simulink model "SF045A_HwAgSysArbn"  (R2013b)
settings: Solver=FixedStepDiscrete  SolverMode=SingleTasking  StartTime=0.0  StopTime=1  FixedStep=.002  RelTol=1e-3
values from neighbouring files (symbols this model uses):
  ARCHGLBPRM_2MILLISEC_SEC_F32 = DataDict.Constant    [SF045A_HwAgSysArbn_DataDict.m]
  ARCHGLBPRM_FLOATZEROTHD_ULS_F32 = DataDict.Constant    [SF045A_HwAgSysArbn_DataDict.m]
  ARCHGLBPRM_PIOVER180_ULS_F32 = DataDict.Constant    [SF045A_HwAgSysArbn_DataDict.m]
  CNVSECTOCNT_ULS_U32 = DataDict.Constant    [SF045A_HwAgSysArbn_DataDict.m]
  CNVTOMILLISEC_MILLISECPERCNT_F32 = DataDict.Constant    [SF045A_HwAgSysArbn_DataDict.m]
  FltInj_f32 = DataDict.Client    [SF045A_HwAgSysArbn_DataDict.m]
  FLTINJ_HWAGSYSARBN_HWAG = DataDict.Constant    [SF045A_HwAgSysArbn_DataDict.m]
  FLTINJ_HWAGSYSARBN_SERLCOMHWAG = DataDict.Constant    [SF045A_HwAgSysArbn_DataDict.m]
  HwAgCorrlnFlt = DataDict.NTC    [SF045A_HwAgSysArbn_DataDict.m]
  HwAgSnsrlsThdExcdd = DataDict.NTC    [SF045A_HwAgSysArbn_DataDict.m]
  HwAgSysArbnHwAgConf1Snsr = DataDict.Calibration    [SF045A_HwAgSysArbn_DataDict.m]
  HwAgSysArbnHwAgConf2Snsr = DataDict.Calibration    [SF045A_HwAgSysArbn_DataDict.m]
  HwAgSysArbnHwAgConfNoSnsr = DataDict.Calibration    [SF045A_HwAgSysArbn_DataDict.m]
  HwAgSysArbnHwAgCorrdCorrlnThd = DataDict.Calibration    [SF045A_HwAgSysArbn_DataDict.m]
  HwAgSysArbnHwAgCorrlnFailDebStep = DataDict.Calibration    [SF045A_HwAgSysArbn_DataDict.m]
  HwAgSysArbnHwAgCorrlnPassDebStep = DataDict.Calibration    [SF045A_HwAgSysArbn_DataDict.m]
  HwAgSysArbnHwAgCorrlnRng = DataDict.Calibration    [SF045A_HwAgSysArbn_DataDict.m]
  HwAgSysArbnHwAgSlewRate = DataDict.Calibration    [SF045A_HwAgSysArbn_DataDict.m]
  HwAgSysArbnHwAgSnsrlsCorrlnThd = DataDict.Calibration    [SF045A_HwAgSysArbn_DataDict.m]
  HwAgSysArbnHwAgSnsrlsKineThd = DataDict.Calibration    [SF045A_HwAgSysArbn_DataDict.m]
  HwAgSysArbnHwAgToMotAgCorrlnElpdTiLim = DataDict.Calibration    [SF045A_HwAgSysArbn_DataDict.m]
  HwAgSysArbnSerlComHwAgCorrdConf = DataDict.Calibration    [SF045A_HwAgSysArbn_DataDict.m]
  HwAgSysArbnSerlComHwAgSnsrlsConf = DataDict.Calibration    [SF045A_HwAgSysArbn_DataDict.m]
  HwAgSysArbnSlewRateTmr = DataDict.Calibration    [SF045A_HwAgSysArbn_DataDict.m]
  HWAGTHD_ULS_FLOAT32 = DataDict.Constant    [SF045A_HwAgSysArbn_DataDict.m]
  INVLDSRC_CNT_S08 = DataDict.Constant    [SF045A_HwAgSysArbn_DataDict.m]
  LRGSLEW_HWDEGPERSEC_F32 = DataDict.Constant    [SF045A_HwAgSysArbn_DataDict.m]
  NODEBSTEP_CNT_U16 = DataDict.Constant    [SF045A_HwAgSysArbn_DataDict.m]
  SLEWINPROGS_CNT_LGC = DataDict.Constant    [SF045A_HwAgSysArbn_DataDict.m]
  SLEWNOTINPROGS_CNT_LGC = DataDict.Constant    [SF045A_HwAgSysArbn_DataDict.m]
  SNSRDATASRCSELD_CNT_S08 = DataDict.Constant    [SF045A_HwAgSysArbn_DataDict.m]
  SNSRLSDATASRCSELD_CNT_S08 = DataDict.Constant    [SF045A_HwAgSysArbn_DataDict.m]
  SysGlbPrmSysKineRat = DataDict.ImprtdCal    [SF045A_HwAgSysArbn_DataDict.m]
  SysGlbPrmTorsBarStfn = DataDict.ImprtdCal    [SF045A_HwAgSysArbn_DataDict.m]
  ZEROTMR_MILLISEC_F32 = DataDict.Constant    [SF045A_HwAgSysArbn_DataDict.m]
undefined symbols (not defined in the file or in its folder): NtcSts1
libraries: NxtrLim x11, simulink x6, NxtrAbslt x6, Fil x3, autosarlib x2
(part 4 of 6)

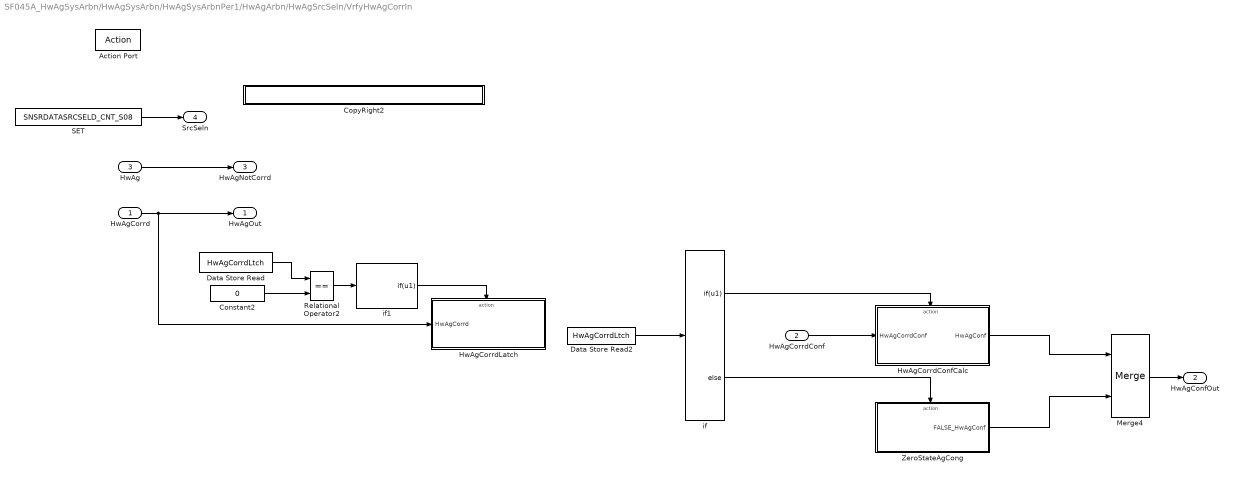
== system SF045A_HwAgSysArbn/HwAgSysArbn/HwAgSysArbnPer1/HwAgArbn/HwAgSrcSeln/VrfyHwAgCorrln ==
  HwAgCorrd : Inport
  HwAgCorrdConf : Inport  Port=2
  HwAg : Inport  Port=3
  Action Port : ActionPort  ActionType=then
  Constant2 : Constant  RequirementInfo={} %GIDa_6d460884_eb57_4a18_b5a0_8df804c20e72  Value=0  OutDataTypeStr=boolean
  CopyRight2 : Subsystem  Description=|  mask(Copyright Information){none=on}
      | Copyright info block.                                               
      |                                                                     
      | Place copyright information at the top of every subsystem in design.
      mask prompts: none "No parameters"
      mask help: Place copyright information at the top of every subsystem in design.
      mask Display:
      | NxtrConf = 'Nexteer Confidential';
      | 
      | sys = bdroot; %handle for the current model ("system")
      | first = get_param(sys,'Created');
      | first = first(end-3:end);  %year is last four digits
      | 
      | last = get_param(sys,'LastModifiedDate');
      | if isempty(last)
      |     last = datestr(now,'yyyy');
      | else
      |     last = last(end-3:end);
      | end
      | 
      | if strcmp(first,last)
      |     fprintf('%s -- Copyright %s Nexteer',NxtrConf,first)
      | else
      |     fprintf('%s -- %s%s- %s Nexteer',NxtrConf,char(169),first,last)
      | end
  Data Store Read : DataStoreRead  RequirementInfo="{'linktype_rmi_doors' '00012ce0 (/E-STEER Core/SubSystem Specifications/Application Functions - EA4/SF045A Handwheel Angle System Arbitration)' '#SF045A_137' 'true' 'REQ:  SF045A_137' '' } %GIDa_194e0ab0_9977_4834_b3f7_b4363b23e19d"  Priority=1  DataStoreName=HwAgCorrdLtch
      settings: AttributesFormatString=Priority%<priority>
  Data Store Read2 : DataStoreRead  RequirementInfo={} %GIDa_535fb5ef_e4a1_4c16_a074_9bb7e8df7af0  Priority=3  DataStoreName=HwAgCorrdLtch
      settings: AttributesFormatString=Priority%<priority>
  HwAgCorrdConfCalc : Subsystem  RequirementInfo="{'linktype_rmi_doors' '00012ce0 (/E-STEER Core/SubSystem Specifications/Application Functions - EA4/SF045A Handwheel Angle System Arbitration)' '#SF045A_143' 'true' 'REQ:  SF045A_143' '' } %GIDa_a84d203b_e366_4371_b9d3_fcddeb517755"  TreatAsAtomicUnit=on
  HwAgCorrdLatch : Subsystem  RequirementInfo="{'linktype_rmi_doors' '00012ce0 (/E-STEER Core/SubSystem Specifications/Application Functions - EA4/SF045A Handwheel Angle System Arbitration)' '#SF045A_142' 'true' 'REQ:  SF045A_142' '' } %GIDa_ab6e831f_d956_473f_8c78_8f53a50bb366"  TreatAsAtomicUnit=on
  Merge4 : Merge  RequirementInfo="{'linktype_rmi_doors' '00012ce0 (/E-STEER Core/SubSystem Specifications/Application Functions - EA4/SF045A Handwheel Angle System Arbitration)' '#SF045A_143' 'true' 'REQ:  SF045A_143' '' ; 'linktype_rmi_doors' '00012ce0 (/E-STEER Core/SubSystem Specifications/Application Functions - EA4/SF045A Handwheel Angle System Arbitration)' '#SF045A_144' 'true' 'REQ:  SF045A_144' '' } %GIDa_b0bab756_8967_46e8_af28_b116f083f0b6"
  Relational Operator2 : RelationalOperator  RequirementInfo={} %GIDa_95e6dac5_bd55_489b_9cc0_b27c478194ec  Operator===  OutDataTypeStr=boolean
  SET : Constant  Value=SNSRDATASRCSELD_CNT_S08
  ZeroStateAgCong : Subsystem  RequirementInfo="{'linktype_rmi_doors' '00012ce0 (/E-STEER Core/SubSystem Specifications/Application Functions - EA4/SF045A Handwheel Angle System Arbitration)' '#SF045A_144' 'true' 'REQ:  SF045A_144' '' } %GIDa_147c3664_39c2_4941_af40_1c56d56f150e"  TreatAsAtomicUnit=on
  if : If  RequirementInfo={} %GIDa_fd8cff81_1f47_4227_b831_50dd22e8a047  IfExpression=u1
  if1 : If  RequirementInfo={} %GIDa_17c9a915_b2cf_43c8_a6ee_d6c1fe1a00d4  IfExpression=u1  ShowElse=off
  HwAgOut : Outport
  HwAgConfOut : Outport  Port=2
  "HwAgNotCorrd " : Outport  Port=3
  SrcSeln : Outport  Port=4
  wires:
  HwAg/1 -> "HwAgNotCorrd "/1
  SET/1 -> SrcSeln/1
  HwAgCorrdConf/1 -> HwAgCorrdConfCalc/1(HwAgCorrdConf)
  Merge4/1 -> HwAgConfOut/1
  Data Store Read/1 -> Relational Operator2/1
  Constant2/1 -> Relational Operator2/2
  Data Store Read2/1 -> if/1
  if/2 -> ZeroStateAgCong/Action
  ZeroStateAgCong/1(FALSE_HwAgConf) -> Merge4/2
  if/1 -> HwAgCorrdConfCalc/Action
  HwAgCorrdConfCalc/1(HwAgConf) -> Merge4/1
  HwAgCorrd/1 -> HwAgCorrdLatch/1(HwAgCorrd), HwAgOut/1
  Relational Operator2/1 -> if1/1
  if1/1 -> HwAgCorrdLatch/Action

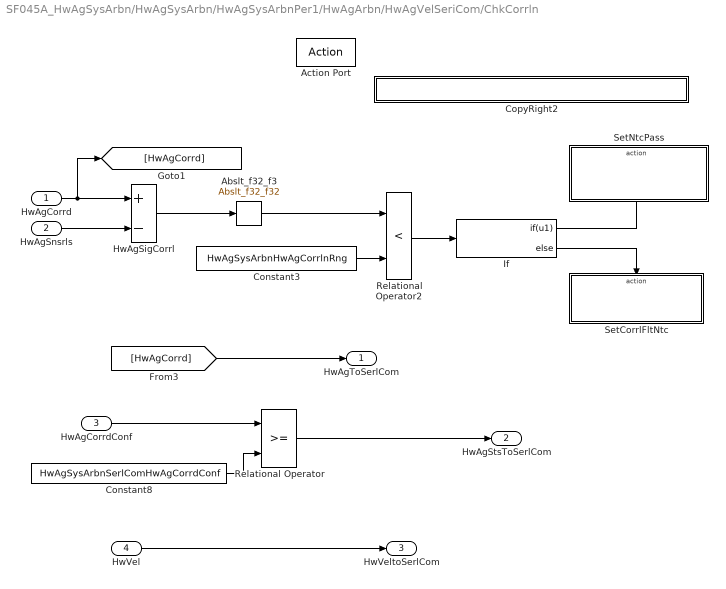
== system SF045A_HwAgSysArbn/HwAgSysArbn/HwAgSysArbnPer1/HwAgArbn/HwAgVelSeriCom/ChkCorrln ==
  HwAgCorrd : Inport
  HwAgSnsrls : Inport  Port=2
  HwAgCorrdConf : Inport  Port=3
  HwVel : Inport  Port=4
  Action Port : ActionPort  ActionType=then
  Abslt_f32_f3 : NxtrAbslt/Abslt_f32_f32  RequirementInfo={} %GIDa_00167e91_613e_4759_885d_9314db63fdd0  SFunctionSpec=single y1 = Abslt_f32_f32(single u1)
      settings: AttributesFormatString=%<Name>
  Constant3 : Constant  RequirementInfo={} %GIDa_be4a7688_2be7_4fe3_8e3d_8bacae0f8621  Value=HwAgSysArbnHwAgCorrlnRng
  Constant8 : Constant  RequirementInfo={} %GIDa_01f8480a_5c21_4e31_ac39_b28c91927747  Value=HwAgSysArbnSerlComHwAgCorrdConf
  CopyRight2 : Subsystem  Description=|  mask(Copyright Information){none=on}
      | Copyright info block.                                               
      |                                                                     
      | Place copyright information at the top of every subsystem in design.
      mask prompts: none "No parameters"
      mask help: Place copyright information at the top of every subsystem in design.
      mask Display:
      | NxtrConf = 'Nexteer Confidential';
      | 
      | sys = bdroot; %handle for the current model ("system")
      | first = get_param(sys,'Created');
      | first = first(end-3:end);  %year is last four digits
      | 
      | last = get_param(sys,'LastModifiedDate');
      | if isempty(last)
      |     last = datestr(now,'yyyy');
      | else
      |     last = last(end-3:end);
      | end
      | 
      | if strcmp(first,last)
      |     fprintf('%s -- Copyright %s Nexteer',NxtrConf,first)
      | else
      |     fprintf('%s -- %s%s- %s Nexteer',NxtrConf,char(169),first,last)
      | end
  HwAgSigCorrl : Sum  RequirementInfo="{'linktype_rmi_doors' '00012ce0 (/E-STEER Core/SubSystem Specifications/Application Functions - EA4/SF045A Handwheel Angle System Arbitration)' '#SF045A_105' 'true' 'REQ:  SF045A_105' '' } %GIDa_a5ccc499_f9e1_47ad_be00_f3d80d727547"  Inputs=+-
  If : If  IfExpression=u1
  Relational Operator : RelationalOperator  RequirementInfo="{'linktype_rmi_doors' '00012ce0 (/E-STEER Core/SubSystem Specifications/Application Functions - EA4/SF045A Handwheel Angle System Arbitration)' '#SF045A_87' 'true' 'REQ:  SF045A_87' '' } %GIDa_d7bb18e9_c0e4_41eb_b2f7_98e90d887605"  OutDataTypeStr=boolean
  Relational Operator2 : RelationalOperator  RequirementInfo="{'linktype_rmi_doors' '00012ce0 (/E-STEER Core/SubSystem Specifications/Application Functions - EA4/SF045A Handwheel Angle System Arbitration)' '#SF045A_105' 'true' 'REQ:  SF045A_105' '' } %GIDa_d5b01a50_0204_46bb_9aa8_dacdb52ec4dd"  Operator=<  OutDataTypeStr=boolean
  SetCorrlFltNtc : Subsystem  RequirementInfo="{'linktype_rmi_doors' '00012ce0 (/E-STEER Core/SubSystem Specifications/Application Functions - EA4/SF045A Handwheel Angle System Arbitration)' '#SF045A_119' 'true' 'REQ:  SF045A_119' '' ; 'linktype_rmi_doors' '00012ce0 (/E-STEER Core/SubSystem Specifications/Application Functions - EA4/SF045A Handwheel Angle System Arbitration)' '#SF045A_102' 'true' 'REQ:  SF045A_102' '' } %GIDa_ccc8f525_72d3_4104_894c_6ee731a3d477"  TreatAsAtomicUnit=on
  SetNtcPass : Subsystem  RequirementInfo="{'linktype_rmi_doors' '00012ce0 (/E-STEER Core/SubSystem Specifications/Application Functions - EA4/SF045A Handwheel Angle System Arbitration)' '#SF045A_118' 'true' 'REQ:  SF045A_118' '' ; 'linktype_rmi_doors' '00012ce0 (/E-STEER Core/SubSystem Specifications/Application Functions - EA4/SF045A Handwheel Angle System Arbitration)' '#SF045A_100' 'true' 'REQ:  SF045A_100' '' } %GIDa_426febc7_a9ce_4f92_8b0a_0ab3cd00c4a5"  TreatAsAtomicUnit=on
  HwAgToSerlCom : Outport
  HwAgStsToSerlCom : Outport  Port=2
  HwVeltoSerlCom : Outport  Port=3
  wires:
  Constant3/1 -> Relational Operator2/2
  Relational Operator2/1 -> If/1
  If/1 -> SetNtcPass/Action
  If/2 -> SetCorrlFltNtc/Action
  Abslt_f32_f3/1 -> Relational Operator2/1
  HwAgCorrd/1 -> [HwAgCorrd], HwAgSigCorrl/1
  HwAgSnsrls/1 -> HwAgSigCorrl/2
  HwAgSigCorrl/1 -> Abslt_f32_f3/1
  [HwAgCorrd] -> HwAgToSerlCom/1
  Constant8/1 -> Relational Operator/2
  Relational Operator/1 -> HwAgStsToSerlCom/1
  HwAgCorrdConf/1 -> Relational Operator/1
  HwVel/1 -> HwVeltoSerlCom/1

== system SF045A_HwAgSysArbn/HwAgSysArbn/HwAgSysArbnPer1/HwAgArbn/HwAgVelSeriCom/CopyRight2 ==

== system SF045A_HwAgSysArbn/HwAgSysArbn/HwAgSysArbnPer1/HwAgArbn/HwAgVelSeriCom/NoHwAgDataToSerlCom ==
  Action Port : ActionPort  ActionType=else
  Constant1 : Constant  RequirementInfo={} %GIDa_a02b812a_5bb2_461f_ace0_8988f08fab8d  Value=0  OutDataTypeStr=single
      settings: AttributesFormatString=%<OutDataTypeStr>
  Constant2 : Constant  RequirementInfo={} %GIDa_f844a0a3_dc21_41b3_ba0d_059082f88489  Value=0  OutDataTypeStr=single
      settings: AttributesFormatString=%<OutDataTypeStr>
  Constant3 : Constant  RequirementInfo={} %GIDa_2bc85182_26c7_4711_9325_d200604b7f8e  Value=0  OutDataTypeStr=boolean
      settings: AttributesFormatString=%<OutDataTypeStr>
  Constant4 : Constant  RequirementInfo={} %GIDa_61722fb7_d0d1_48a0_9b35_b7bb428fb489  Value=false  OutDataTypeStr=boolean
      settings: AttributesFormatString=%<OutDataTypeStr>
  CopyRight2 : Subsystem  Description=|  mask(Copyright Information){none=on}
      | Copyright info block.                                               
      |                                                                     
      | Place copyright information at the top of every subsystem in design.
      mask prompts: none "No parameters"
      mask help: Place copyright information at the top of every subsystem in design.
      mask Display:
      | NxtrConf = 'Nexteer Confidential';
      | 
      | sys = bdroot; %handle for the current model ("system")
      | first = get_param(sys,'Created');
      | first = first(end-3:end);  %year is last four digits
      | 
      | last = get_param(sys,'LastModifiedDate');
      | if isempty(last)
      |     last = datestr(now,'yyyy');
      | else
      |     last = last(end-3:end);
      | end
      | 
      | if strcmp(first,last)
      |     fprintf('%s -- Copyright %s Nexteer',NxtrConf,first)
      | else
      |     fprintf('%s -- %s%s- %s Nexteer',NxtrConf,char(169),first,last)
      | end
  Data Store Write1 : DataStoreWrite  RequirementInfo={} %GIDa_e6de61ed_04b3_4d58_aa8c_0cc6c6a7d4ac  DataStoreName=HwAgToMotAgCorrln
  HwAgToSerlCom : Outport  RequirementInfo={} %GIDa_87d34148_265f_40b9_ba05_ef974c74b368
  HwAgStsToSerlCom : Outport  RequirementInfo={} %GIDa_bc4a4d7d_6692_4a24_9b5a_dae1ee87d15a  Port=2
  HwVelToSerlCom : Outport  RequirementInfo={} %GIDa_292181ae_ff5a_44a7_9b1e_cbcb900e661b  Port=3
  wires:
  Constant3/1 -> HwAgStsToSerlCom/1
  Constant1/1 -> HwAgToSerlCom/1
  Constant4/1 -> Data Store Write1/1
  Constant2/1 -> HwVelToSerlCom/1

== system SF045A_HwAgSysArbn/HwAgSysArbn/HwAgSysArbnPer1/HwAgArbn/HwAgVelSeriCom/SnsrDataToSerlCom ==
  HwAgCorrd : Inport
  HwAgCorrdConf : Inport  Port=2
  HwVel : Inport  Port=3
  Action Port : ActionPort  ActionType=elseif
  Constant4 : Constant  RequirementInfo={} %GIDa_a5c0f91e_a234_41bc_8819_bbc101ae7768  Value=false  OutDataTypeStr=boolean
      settings: AttributesFormatString=%<OutDataTypeStr>
  Constant8 : Constant  RequirementInfo={} %GIDa_2fa74474_72fc_414f_bfbb_6838e73092f3  Value=HwAgSysArbnSerlComHwAgCorrdConf
  CopyRight2 : Subsystem  Description=|  mask(Copyright Information){none=on}
      | Copyright info block.                                               
      |                                                                     
      | Place copyright information at the top of every subsystem in design.
      mask prompts: none "No parameters"
      mask help: Place copyright information at the top of every subsystem in design.
      mask Display:
      | NxtrConf = 'Nexteer Confidential';
      | 
      | sys = bdroot; %handle for the current model ("system")
      | first = get_param(sys,'Created');
      | first = first(end-3:end);  %year is last four digits
      | 
      | last = get_param(sys,'LastModifiedDate');
      | if isempty(last)
      |     last = datestr(now,'yyyy');
      | else
      |     last = last(end-3:end);
      | end
      | 
      | if strcmp(first,last)
      |     fprintf('%s -- Copyright %s Nexteer',NxtrConf,first)
      | else
      |     fprintf('%s -- %s%s- %s Nexteer',NxtrConf,char(169),first,last)
      | end
  Data Store Write1 : DataStoreWrite  RequirementInfo={} %GIDa_7d4d65e4_5bda_40f3_9819_0c867367088e  DataStoreName=HwAgToMotAgCorrln
  Relational Operator : RelationalOperator  RequirementInfo="{'linktype_rmi_doors' '00012ce0 (/E-STEER Core/SubSystem Specifications/Application Functions - EA4/SF045A Handwheel Angle System Arbitration)' '#SF045A_87' 'true' 'REQ:  SF045A_87' '' } %GIDa_0016588c_6b78_4f89_9589_bb8824a4e019"  OutDataTypeStr=boolean
  HwAgToSerlCom : Outport
  HwAgStsToSerlCom : Outport  Port=2
  HwVeltoSerlCom : Outport  Port=3
  wires:
  HwAgCorrd/1 -> HwAgToSerlCom/1
  Constant8/1 -> Relational Operator/2
  Relational Operator/1 -> HwAgStsToSerlCom/1
  HwAgCorrdConf/1 -> Relational Operator/1
  Constant4/1 -> Data Store Write1/1
  HwVel/1 -> HwVeltoSerlCom/1

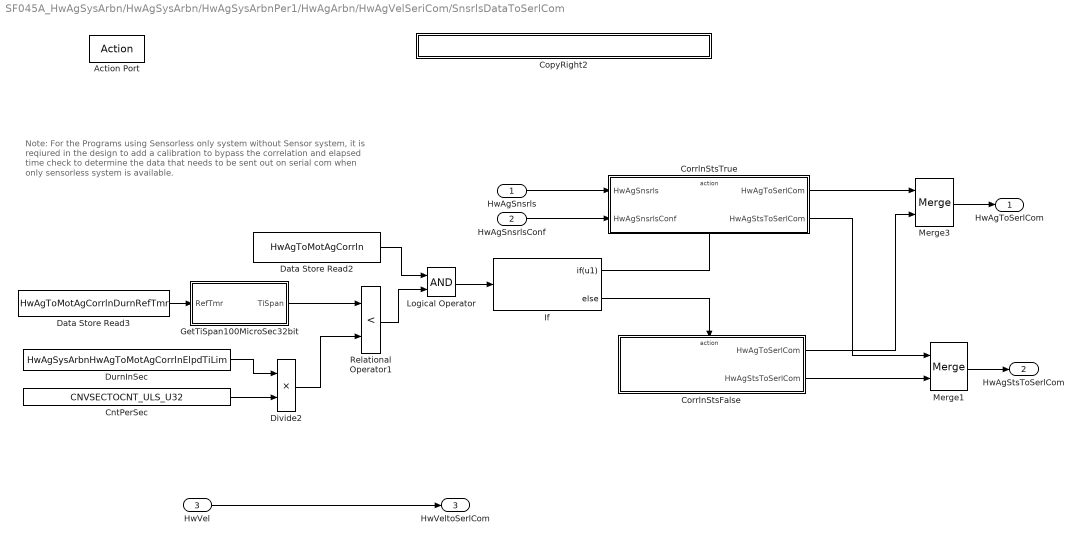
== system SF045A_HwAgSysArbn/HwAgSysArbn/HwAgSysArbnPer1/HwAgArbn/HwAgVelSeriCom/SnsrlsDataToSerlCom ==
  note: Note: For the Programs using Sensorless only system without Sensor system,
      | it is reqiured in the design to add a calibration to bypass the correlation
      | and  elapsed time check to determine the data that needs to be
      | sent out on serial com when only sensorless system is available.
  HwAgSnsrls : Inport
  HwAgSnsrlsConf : Inport  Port=2
  HwVel : Inport  Port=3
  Action Port : ActionPort  ActionType=elseif
  CntPerSec : Constant  RequirementInfo={} %GIDa_6f300a99_6407_4b06_9b16_83ced7363eb6  Value=CNVSECTOCNT_ULS_U32
  CopyRight2 : Subsystem  Description=|  mask(Copyright Information){none=on}
      | Copyright info block.                                               
      |                                                                     
      | Place copyright information at the top of every subsystem in design.
      mask prompts: none "No parameters"
      mask help: Place copyright information at the top of every subsystem in design.
      mask Display:
      | NxtrConf = 'Nexteer Confidential';
      | 
      | sys = bdroot; %handle for the current model ("system")
      | first = get_param(sys,'Created');
      | first = first(end-3:end);  %year is last four digits
      | 
      | last = get_param(sys,'LastModifiedDate');
      | if isempty(last)
      |     last = datestr(now,'yyyy');
      | else
      |     last = last(end-3:end);
      | end
      | 
      | if strcmp(first,last)
      |     fprintf('%s -- Copyright %s Nexteer',NxtrConf,first)
      | else
      |     fprintf('%s -- %s%s- %s Nexteer',NxtrConf,char(169),first,last)
      | end
  CorrlnStsFalse : Subsystem  RequirementInfo="{'linktype_rmi_doors' '00012ce0 (/E-STEER Core/SubSystem Specifications/Application Functions - EA4/SF045A Handwheel Angle System Arbitration)' '#SF045A_88' 'true' 'REQ:  SF045A_88' '' } %GIDa_9aa11952_02dd_4fb1_97aa_6c9f9669e7c8"  TreatAsAtomicUnit=on
  CorrlnStsTrue : Subsystem  RequirementInfo="{'linktype_rmi_doors' '00012ce0 (/E-STEER Core/SubSystem Specifications/Application Functions - EA4/SF045A Handwheel Angle System Arbitration)' '#SF045A_126' 'true' 'REQ:  SF045A_126' '' } %GIDa_c11b99f2_5a6b_481f_87db_34ffecccd82d"  TreatAsAtomicUnit=on
  Data Store Read2 : DataStoreRead  RequirementInfo={} %GIDa_d157e0e2_c646_4139_84ff_d426e3cb2c85  DataStoreName=HwAgToMotAgCorrln
  Data Store Read3 : DataStoreRead  RequirementInfo={} %GIDa_80ea55d1_0217_4e7b_bf4d_fe61b5a75119  DataStoreName=HwAgToMotAgCorrlnDurnRefTmr
  Divide2 : Product  RequirementInfo="{'linktype_rmi_doors' '00012ce0 (/E-STEER Core/SubSystem Specifications/Application Functions - EA4/SF045A Handwheel Angle System Arbitration)' '#SF045A_88' 'true' 'REQ:  SF045A_88' '' } %GIDa_bcb7c231_ed3b_4158_a22f_2ba1135223c3"  Inputs=**
  DurnInSec : Constant  RequirementInfo={} %GIDa_8fdd184e_2623_4630_9833_75dd9914401a  Value=HwAgSysArbnHwAgToMotAgCorrlnElpdTiLim
  GetTiSpan100MicroSec32bit : Subsystem  mask(Timer_GTS){}
      mask help: Used to get the time span between start and current time.
  If : If  RequirementInfo="{'linktype_rmi_doors' '00012ce0 (/E-STEER Core/SubSystem Specifications/Application Functions - EA4/SF045A Handwheel Angle System Arbitration)' '#SF045A_88' 'true' 'REQ:  SF045A_88' '' } %GIDa_f006d63e_e2e6_452a_b329_053a8c87baba"  IfExpression=u1
  Logical Operator : Logic  RequirementInfo="{'linktype_rmi_doors' '00012ce0 (/E-STEER Core/SubSystem Specifications/Application Functions - EA4/SF045A Handwheel Angle System Arbitration)' '#SF045A_88' 'true' 'REQ:  SF045A_88' '' } %GIDa_a7566d14_a88f_4d0f_831f_4ebb74da1490"  AllPortsSameDT=off  OutDataTypeStr=boolean
  Merge1 : Merge  RequirementInfo="{'linktype_rmi_doors' '00012ce0 (/E-STEER Core/SubSystem Specifications/Application Functions - EA4/SF045A Handwheel Angle System Arbitration)' '#SF045A_88' 'true' 'REQ:  SF045A_88' '' } %GIDa_ae9d6315_3d26_4bd0_a0ce_476f62b97700"
  Merge3 : Merge  RequirementInfo="{'linktype_rmi_doors' '00012ce0 (/E-STEER Core/SubSystem Specifications/Application Functions - EA4/SF045A Handwheel Angle System Arbitration)' '#SF045A_88' 'true' 'REQ:  SF045A_88' '' } %GIDa_95cf898e_c41c_48bb_851c_3e79950b385d"
  Relational Operator1 : RelationalOperator  RequirementInfo="{'linktype_rmi_doors' '00012ce0 (/E-STEER Core/SubSystem Specifications/Application Functions - EA4/SF045A Handwheel Angle System Arbitration)' '#SF045A_88' 'true' 'REQ:  SF045A_88' '' } %GIDa_252f9f36_3ba8_4ad5_b5ef_1a270203ec38"  Operator=<  OutDataTypeStr=boolean
  HwAgToSerlCom : Outport  RequirementInfo={} %GIDa_23c32ff2_460d_420f_8ac6_bd591d4df452
  HwAgStsToSerlCom : Outport  RequirementInfo={} %GIDa_51dcb0ad_eafc_44a5_b94c_ae4d6c5ea78f  Port=2
  HwVeltoSerlCom : Outport  Port=3
  wires:
  Logical Operator/1 -> If/1
  If/1 -> CorrlnStsTrue/Action
  If/2 -> CorrlnStsFalse/Action
  HwAgSnsrls/1 -> CorrlnStsTrue/1(HwAgSnsrls)
  HwAgSnsrlsConf/1 -> CorrlnStsTrue/2(HwAgSnsrlsConf)
  Merge1/1 -> HwAgStsToSerlCom/1
  Merge3/1 -> HwAgToSerlCom/1
  CorrlnStsFalse/1(HwAgToSerlCom) -> Merge3/2
  CorrlnStsFalse/2(HwAgStsToSerlCom) -> Merge1/2
  Relational Operator1/1 -> Logical Operator/2
  GetTiSpan100MicroSec32bit/1(TiSpan) -> Relational Operator1/1
  Divide2/1 -> Relational Operator1/2
  CntPerSec/1 -> Divide2/2
  Data Store Read2/1 -> Logical Operator/1
  Data Store Read3/1 -> GetTiSpan100MicroSec32bit/1(RefTmr)
  CorrlnStsTrue/1(HwAgToSerlCom) -> Merge3/1
  CorrlnStsTrue/2(HwAgStsToSerlCom) -> Merge1/1
  DurnInSec/1 -> Divide2/1
  HwVel/1 -> HwVeltoSerlCom/1

== system SF045A_HwAgSysArbn/HwAgSysArbn/HwAgSysArbnPer1/HwAgArbn/TestHwAgSrcChg/ApplyLrgSlew ==
  Action Port : ActionPort  ActionType=else
  Constant1 : Constant  Value=LRGSLEW_HWDEGPERSEC_F32
  Constant3 : Constant  Value=ZEROTMR_MILLISEC_F32
  CopyRight2 : Subsystem  Description=|  mask(Copyright Information){none=on}
      | Copyright info block.                                               
      |                                                                     
      | Place copyright information at the top of every subsystem in design.
      mask prompts: none "No parameters"
      mask help: Place copyright information at the top of every subsystem in design.
      mask Display:
      | NxtrConf = 'Nexteer Confidential';
      | 
      | sys = bdroot; %handle for the current model ("system")
      | first = get_param(sys,'Created');
      | first = first(end-3:end);  %year is last four digits
      | 
      | last = get_param(sys,'LastModifiedDate');
      | if isempty(last)
      |     last = datestr(now,'yyyy');
      | else
      |     last = last(end-3:end);
      | end
      | 
      | if strcmp(first,last)
      |     fprintf('%s -- Copyright %s Nexteer',NxtrConf,first)
      | else
      |     fprintf('%s -- %s%s- %s Nexteer',NxtrConf,char(169),first,last)
      | end
  SlewRate : Outport
  SlewElpdTiLim : Outport  Port=2
  wires:
  Constant1/1 -> SlewRate/1
  Constant3/1 -> SlewElpdTiLim/1

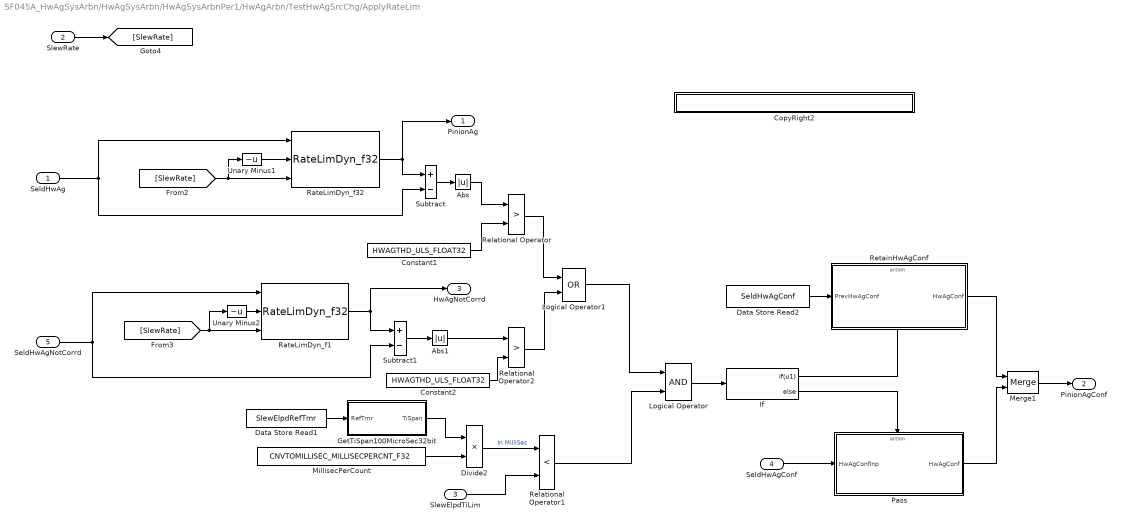
== system SF045A_HwAgSysArbn/HwAgSysArbn/HwAgSysArbnPer1/HwAgArbn/TestHwAgSrcChg/ApplyRateLim ==
  SeldHwAg : Inport  RequirementInfo={} %GIDa_6b4546cd_b9fa_44eb_9405_c24958722829
  SlewRate : Inport  RequirementInfo={} %GIDa_e89af669_bce9_444b_9eca_e0104ba5720b  Port=2
  SlewElpdTiLim : Inport  RequirementInfo={} %GIDa_ab1a8e03_a319_4288_8e98_7e4c6130b5b7  Port=3
  SeldHwAgConf : Inport  Port=4
  SeldHwAgNotCorrd : Inport  RequirementInfo={} %GIDa_1ea6bbf3_7e61_492d_a285_d9a199a276c2  Port=5
  Abs : Abs  RequirementInfo={} %GIDa_7d983b87_bb5e_439f_89a0_e67f0114ec94
  Abs1 : Abs  RequirementInfo={} %GIDa_9bfaa416_c3ce_4cdb_8a15_75e15780b4a4
  Constant1 : Constant  RequirementInfo={} %GIDa_50458eea_d28c_4367_ba5c_179a92a1621e  Value=HWAGTHD_ULS_FLOAT32
  Constant2 : Constant  RequirementInfo={} %GIDa_d8d15a73_ba3f_43c0_b439_3fda6cce7bca  Value=HWAGTHD_ULS_FLOAT32
  CopyRight2 : Subsystem  Description=|  mask(Copyright Information){none=on}
      | Copyright info block.                                               
      |                                                                     
      | Place copyright information at the top of every subsystem in design.
      mask prompts: none "No parameters"
      mask help: Place copyright information at the top of every subsystem in design.
      mask Display:
      | NxtrConf = 'Nexteer Confidential';
      | 
      | sys = bdroot; %handle for the current model ("system")
      | first = get_param(sys,'Created');
      | first = first(end-3:end);  %year is last four digits
      | 
      | last = get_param(sys,'LastModifiedDate');
      | if isempty(last)
      |     last = datestr(now,'yyyy');
      | else
      |     last = last(end-3:end);
      | end
      | 
      | if strcmp(first,last)
      |     fprintf('%s -- Copyright %s Nexteer',NxtrConf,first)
      | else
      |     fprintf('%s -- %s%s- %s Nexteer',NxtrConf,char(169),first,last)
      | end
  Data Store Read1 : DataStoreRead  RequirementInfo="{'linktype_rmi_doors' '00012ce0 (/E-STEER Core/SubSystem Specifications/Application Functions - EA4/SF045A Handwheel Angle System Arbitration)' '#SF045A_78' 'true' 'REQ:  SF045A_78' '' } %GIDa_77d697ad_05a5_4668_ae2b_f296325b8e61"  DataStoreName=SlewElpdRefTmr
  Data Store Read2 : DataStoreRead  RequirementInfo={} %GIDa_9956a642_5465_47c9_b349_65821ff398fe  DataStoreName=SeldHwAgConf
  Divide2 : Product  RequirementInfo="{'linktype_rmi_doors' '00012ce0 (/E-STEER Core/SubSystem Specifications/Application Functions - EA4/SF045A Handwheel Angle System Arbitration)' '#SF045A_78' 'true' 'REQ:  SF045A_78' '' ; 'linktype_rmi_doors' '00012ce0 (/E-STEER Core/SubSystem Specifications/Application Functions - EA4/SF045A Handwheel Angle System Arbitration)' '#SF045A_79' 'true' 'REQ:  SF045A_79' '' } %GIDa_ed53147f_35d8_45a8_a4ed_db5c7ea7a303"  Inputs=**
  GetTiSpan100MicroSec32bit : Subsystem  mask(Timer_GTS){}
      mask help: Used to get the time span between start and current time.
  If : If  RequirementInfo="{'linktype_rmi_doors' '00012ce0 (/E-STEER Core/SubSystem Specifications/Application Functions - EA4/SF045A Handwheel Angle System Arbitration)' '#SF045A_79' 'true' 'REQ:  SF045A_79' '' ; 'linktype_rmi_doors' '00012ce0 (/E-STEER Core/SubSystem Specifications/Application Functions - EA4/SF045A Handwheel Angle System Arbitration)' '#SF045A_78' 'true' 'REQ:  SF045A_78' '' } %GIDa_4eef1f53_1d49_4df6_a935_4c88f948f870"  IfExpression=u1
  Logical Operator : Logic  RequirementInfo="{'linktype_rmi_doors' '00012ce0 (/E-STEER Core/SubSystem Specifications/Application Functions - EA4/SF045A Handwheel Angle System Arbitration)' '#SF045A_78' 'true' 'REQ:  SF045A_78' '' ; 'linktype_rmi_doors' '00012ce0 (/E-STEER Core/SubSystem Specifications/Application Functions - EA4/SF045A Handwheel Angle System Arbitration)' '#SF045A_79' 'true' 'REQ:  SF045A_79' '' } %GIDa_c8d83738_7f44_43f2_b0fc_adf7f32547c5"  AllPortsSameDT=off  OutDataTypeStr=boolean
  Logical Operator1 : Logic  RequirementInfo="{'linktype_rmi_doors' '00012ce0 (/E-STEER Core/SubSystem Specifications/Application Functions - EA4/SF045A Handwheel Angle System Arbitration)' '#SF045A_78' 'true' 'REQ:  SF045A_78' '' ; 'linktype_rmi_doors' '00012ce0 (/E-STEER Core/SubSystem Specifications/Application Functions - EA4/SF045A Handwheel Angle System Arbitration)' '#SF045A_79' 'true' 'REQ:  SF045A_79' '' } %GIDa_d1bf9721_754c_4a6e_860d_9591702c7ba7"  Operator=OR  AllPortsSameDT=off  OutDataTypeStr=boolean
  Merge1 : Merge
  MillisecPerCount : Constant  RequirementInfo={} %GIDa_2cd47510_639f_4aee_9025_bd1fad54e509  Value=CNVTOMILLISEC_MILLISECPERCNT_F32
  Pass : Subsystem  RequirementInfo="{'linktype_rmi_doors' '00012ce0 (/E-STEER Core/SubSystem Specifications/Application Functions - EA4/SF045A Handwheel Angle System Arbitration)' '#SF045A_79' 'true' 'REQ:  SF045A_79' '' ; 'linktype_rmi_doors' '00012ce0 (/E-STEER Core/SubSystem Specifications/Application Functions - EA4/SF045A Handwheel Angle System Arbitration)' '#SF045A_78' 'true' 'REQ:  SF045A_78' '' } %GIDa_77e98a5c_29d3_4b88_a338_2bbaec01eb13"  TreatAsAtomicUnit=on
  RateLimDyn_f1 : NxtrLim/RateLimDyn_f32  RequirementInfo="{'linktype_rmi_doors' '00012ce0 (/E-STEER Core/SubSystem Specifications/Application Functions - EA4/SF045A Handwheel Angle System Arbitration)' '#SF045A_77' 'true' 'REQ:  SF045A_77' '' ; 'linktype_rmi_doors' '00012ce0 (/E-STEER Core/SubSystem Specifications/Application Functions - EA4/SF045A Handwheel Angle System Arbitration)' '#SF045A_78' 'true' 'REQ:  SF045A_78' '' ; 'linktype_rmi_doors' '00012ce0 (/E-STEER Core/SubSystem Specifications/Application Functions - EA4/SF045A Handwheel Angle System Arbitration)' '#SF045A_79' 'true' 'REQ:  SF045A_79' '' } %GIDa_d8cc7331_fcd2_4584_8cbe_e7a334d958ff"  StVar=PrevHwAgNotCorrd  Ts=ARCHGLBPRM_2MILLISEC_SEC_F32
      settings: AttributesFormatString=StVar: %<StVar>
  RateLimDyn_f32 : NxtrLim/RateLimDyn_f32  RequirementInfo="{'linktype_rmi_doors' '00012ce0 (/E-STEER Core/SubSystem Specifications/Application Functions - EA4/SF045A Handwheel Angle System Arbitration)' '#SF045A_77' 'true' 'REQ:  SF045A_77' '' ; 'linktype_rmi_doors' '00012ce0 (/E-STEER Core/SubSystem Specifications/Application Functions - EA4/SF045A Handwheel Angle System Arbitration)' '#SF045A_78' 'true' 'REQ:  SF045A_78' '' ; 'linktype_rmi_doors' '00012ce0 (/E-STEER Core/SubSystem Specifications/Application Functions - EA4/SF045A Handwheel Angle System Arbitration)' '#SF045A_79' 'true' 'REQ:  SF045A_79' '' } %GIDa_4ac77c27_e05a_467d_a0f8_fb077551b667"  StVar=PrevSeldHwAg  Ts=ARCHGLBPRM_2MILLISEC_SEC_F32
      settings: AttributesFormatString=StVar: %<StVar>
  Relational Operator : RelationalOperator  RequirementInfo="{'linktype_rmi_doors' '00012ce0 (/E-STEER Core/SubSystem Specifications/Application Functions - EA4/SF045A Handwheel Angle System Arbitration)' '#SF045A_78' 'true' 'REQ:  SF045A_78' '' ; 'linktype_rmi_doors' '00012ce0 (/E-STEER Core/SubSystem Specifications/Application Functions - EA4/SF045A Handwheel Angle System Arbitration)' '#SF045A_79' 'true' 'REQ:  SF045A_79' '' } %GIDa_07caeafa_f744_4d0d_a6ff_b458d6b21ebd"  Operator=>  OutDataTypeStr=boolean
  Relational Operator1 : RelationalOperator  RequirementInfo="{'linktype_rmi_doors' '00012ce0 (/E-STEER Core/SubSystem Specifications/Application Functions - EA4/SF045A Handwheel Angle System Arbitration)' '#SF045A_78' 'true' 'REQ:  SF045A_78' '' ; 'linktype_rmi_doors' '00012ce0 (/E-STEER Core/SubSystem Specifications/Application Functions - EA4/SF045A Handwheel Angle System Arbitration)' '#SF045A_79' 'true' 'REQ:  SF045A_79' '' } %GIDa_77c8a915_3a05_47cb_87ba_d481702a8bd0"  Operator=<  OutDataTypeStr=boolean
  Relational Operator2 : RelationalOperator  RequirementInfo="{'linktype_rmi_doors' '00012ce0 (/E-STEER Core/SubSystem Specifications/Application Functions - EA4/SF045A Handwheel Angle System Arbitration)' '#SF045A_78' 'true' 'REQ:  SF045A_78' '' ; 'linktype_rmi_doors' '00012ce0 (/E-STEER Core/SubSystem Specifications/Application Functions - EA4/SF045A Handwheel Angle System Arbitration)' '#SF045A_79' 'true' 'REQ:  SF045A_79' '' } %GIDa_7510a5f7_b9a6_46ba_99c6_8dfe823e8b23"  Operator=>  OutDataTypeStr=boolean
  RetainHwAgConf : Subsystem  RequirementInfo="{'linktype_rmi_doors' '00012ce0 (/E-STEER Core/SubSystem Specifications/Application Functions - EA4/SF045A Handwheel Angle System Arbitration)' '#SF045A_79' 'true' 'REQ:  SF045A_79' '' ; 'linktype_rmi_doors' '00012ce0 (/E-STEER Core/SubSystem Specifications/Application Functions - EA4/SF045A Handwheel Angle System Arbitration)' '#SF045A_78' 'true' 'REQ:  SF045A_78' '' } %GIDa_e4bdba54_4d12_4955_aae1_99c88c18e07d"  TreatAsAtomicUnit=on
  Subtract : Sum  RequirementInfo="{'linktype_rmi_doors' '00012ce0 (/E-STEER Core/SubSystem Specifications/Application Functions - EA4/SF045A Handwheel Angle System Arbitration)' '#SF045A_77' 'true' 'REQ:  SF045A_77' '' ; 'linktype_rmi_doors' '00012ce0 (/E-STEER Core/SubSystem Specifications/Application Functions - EA4/SF045A Handwheel Angle System Arbitration)' '#SF045A_78' 'true' 'REQ:  SF045A_78' '' ; 'linktype_rmi_doors' '00012ce0 (/E-STEER Core/SubSystem Specifications/Application Functions - EA4/SF045A Handwheel Angle System Arbitration)' '#SF045A_79' 'true' 'REQ:  SF045A_79' '' } %GIDa_7a52a723_ac79_4275_a745_5e82ab096a47"  Inputs=+-
  Subtract1 : Sum  RequirementInfo="{'linktype_rmi_doors' '00012ce0 (/E-STEER Core/SubSystem Specifications/Application Functions - EA4/SF045A Handwheel Angle System Arbitration)' '#SF045A_77' 'true' 'REQ:  SF045A_77' '' ; 'linktype_rmi_doors' '00012ce0 (/E-STEER Core/SubSystem Specifications/Application Functions - EA4/SF045A Handwheel Angle System Arbitration)' '#SF045A_78' 'true' 'REQ:  SF045A_78' '' ; 'linktype_rmi_doors' '00012ce0 (/E-STEER Core/SubSystem Specifications/Application Functions - EA4/SF045A Handwheel Angle System Arbitration)' '#SF045A_79' 'true' 'REQ:  SF045A_79' '' } %GIDa_f62acac5_e933_40cc_8219_5dbf1525909e"  Inputs=+-
  Unary Minus1 : UnaryMinus  RequirementInfo={} %GIDa_54f875f1_ed7b_436d_a76d_5073f7d76cd1
  Unary Minus2 : UnaryMinus  RequirementInfo={} %GIDa_7a98fa4a_a943_4e34_9c77_88b41fead954
  PinionAg : Outport  RequirementInfo={} %GIDa_fabb7919_865f_4124_8835_c8e83112638a
  PinionAgConf : Outport  Port=2
  HwAgNotCorrd : Outport  RequirementInfo={} %GIDa_e813e286_65b1_4ce5_8ae8_120b40ef2b4d  Port=3
  wires:
  SeldHwAg/1 -> Subtract/2, RateLimDyn_f32/1
  [SlewRate] -> Unary Minus1/1, RateLimDyn_f32/3
  Unary Minus1/1 -> RateLimDyn_f32/2
  Subtract/1 -> Abs/1
  Abs/1 -> Relational Operator/1
  Constant1/1 -> Relational Operator/2
  Relational Operator1/1 -> Logical Operator/2
  Logical Operator/1 -> If/1
  If/1 -> RetainHwAgConf/Action
  If/2 -> Pass/Action
  Data Store Read2/1 -> RetainHwAgConf/1(PrevHwAgConf)
  SeldHwAgConf/1 -> Pass/1(HwAgConfInp)
  Merge1/1 -> PinionAgConf/1
  RetainHwAgConf/1("HwAgConf ") -> Merge1/1
  Pass/1("HwAgConf ") -> Merge1/2
  Divide2/1 -> Relational Operator1/1  "In MilliSec"
  SlewElpdTiLim/1 -> Relational Operator1/2
  Data Store Read1/1 -> GetTiSpan100MicroSec32bit/1(RefTmr)
  RateLimDyn_f32/1 -> PinionAg/1, Subtract/1
  GetTiSpan100MicroSec32bit/1(TiSpan) -> Divide2/1
  MillisecPerCount/1 -> Divide2/2
  SlewRate/1 -> [SlewRate]
  [SlewRate] -> Unary Minus2/1, RateLimDyn_f1/3
  Unary Minus2/1 -> RateLimDyn_f1/2
  SeldHwAgNotCorrd/1 -> Subtract1/2, RateLimDyn_f1/1
  Subtract1/1 -> Abs1/1
  Abs1/1 -> Relational Operator2/1
  Constant2/1 -> Relational Operator2/2
  RateLimDyn_f1/1 -> HwAgNotCorrd/1, Subtract1/1
  Relational Operator/1 -> Logical Operator1/1
  Relational Operator2/1 -> Logical Operator1/2
  Logical Operator1/1 -> Logical Operator/1

== system SF045A_HwAgSysArbn/HwAgSysArbn/HwAgSysArbnPer1/HwAgArbn/TestHwAgSrcChg/CopyRight2 ==

== system SF045A_HwAgSysArbn/HwAgSysArbn/HwAgSysArbnPer1/HwAgArbn/TestHwAgSrcChg/RetainSlewRate ==
  Action Port : ActionPort  ActionType=elseif
  Constant2 : Constant  RequirementInfo={} %GIDa_bf13fa7c_3573_4b03_80b9_2ede92d79281  Value=HwAgSysArbnHwAgSlewRate
  Constant4 : Constant  RequirementInfo={} %GIDa_1b593459_32c3_40e5_a98f_c3442c4f19f7  Value=HwAgSysArbnSlewRateTmr
  CopyRight2 : Subsystem  Description=|  mask(Copyright Information){none=on}
      | Copyright info block.                                               
      |                                                                     
      | Place copyright information at the top of every subsystem in design.
      mask prompts: none "No parameters"
      mask help: Place copyright information at the top of every subsystem in design.
      mask Display:
      | NxtrConf = 'Nexteer Confidential';
      | 
      | sys = bdroot; %handle for the current model ("system")
      | first = get_param(sys,'Created');
      | first = first(end-3:end);  %year is last four digits
      | 
      | last = get_param(sys,'LastModifiedDate');
      | if isempty(last)
      |     last = datestr(now,'yyyy');
      | else
      |     last = last(end-3:end);
      | end
      | 
      | if strcmp(first,last)
      |     fprintf('%s -- Copyright %s Nexteer',NxtrConf,first)
      | else
      |     fprintf('%s -- %s%s- %s Nexteer',NxtrConf,char(169),first,last)
      | end
  SlewRate : Outport
  "SlewElpdTiLim " : Outport  Port=2
  wires:
  Constant4/1 -> "SlewElpdTiLim "/1
  Constant2/1 -> SlewRate/1

== system SF045A_HwAgSysArbn/HwAgSysArbn/HwAgSysArbnPer1/HwAgArbn/TestHwAgSrcChg/SetSlewRate ==
  PrsntSrcSeln : Inport  RequirementInfo={} %GIDa_5a1e18eb_9d9e_4825_b5bf_f6dd4468d44e
  Action Port : ActionPort  ActionType=then
  Constant5 : Constant  RequirementInfo={} %GIDa_0f131a30_9c8f_43f4_ab96_9072110bb0ad  Value=HwAgSysArbnHwAgSlewRate
  Constant6 : Constant  RequirementInfo={} %GIDa_23f6532f_1613_463e_bc86_2d4195bd1ea1  Value=HwAgSysArbnSlewRateTmr
  CopyRight2 : Subsystem  Description=|  mask(Copyright Information){none=on}
      | Copyright info block.                                               
      |                                                                     
      | Place copyright information at the top of every subsystem in design.
      mask prompts: none "No parameters"
      mask help: Place copyright information at the top of every subsystem in design.
      mask Display:
      | NxtrConf = 'Nexteer Confidential';
      | 
      | sys = bdroot; %handle for the current model ("system")
      | first = get_param(sys,'Created');
      | first = first(end-3:end);  %year is last four digits
      | 
      | last = get_param(sys,'LastModifiedDate');
      | if isempty(last)
      |     last = datestr(now,'yyyy');
      | else
      |     last = last(end-3:end);
      | end
      | 
      | if strcmp(first,last)
      |     fprintf('%s -- Copyright %s Nexteer',NxtrConf,first)
      | else
      |     fprintf('%s -- %s%s- %s Nexteer',NxtrConf,char(169),first,last)
      | end
  Data Store Read2 : DataStoreRead  RequirementInfo={} %GIDa_afd0f656_3550_4018_ad78_b5d08cf73971  DataStoreName=PrevPinionAgConf
  Data Store Write2 : DataStoreWrite  RequirementInfo={} %GIDa_580680a2_326c_41c8_8061_632772c4720f  DataStoreName=SeldHwAgConf
  Data Store Write3 : DataStoreWrite  RequirementInfo={} %GIDa_a0eb0094_cd50_47f8_9b0e_d3620d4ed205  DataStoreName=SlewElpdRefTmr
  Data Store Write6 : DataStoreWrite  RequirementInfo={} %GIDa_5d7c1c12_4ced_477e_835f_5a449bab2d82  DataStoreName=PrevSrcSeln
  GetRefTmr100MicroSec32bit : Subsystem  RequirementInfo={} %GIDa_0c4a519d_41c1_450f_a5ea_c9a6a8594b5f
  SlewRate : Outport
  "SlewElpdTiLim " : Outport  Port=2
  wires:
  Data Store Read2/1 -> Data Store Write2/1
  PrsntSrcSeln/1 -> Data Store Write6/1
  GetRefTmr100MicroSec32bit/1(RefTmr) -> Data Store Write3/1
  Constant5/1 -> SlewRate/1
  Constant6/1 -> "SlewElpdTiLim "/1

== system SF045A_HwAgSysArbn/HwAgSysArbn/HwAgSysArbnPer1/HwAgArbn/VldtSnsrlsData/CopyRight2 ==

== system SF045A_HwAgSysArbn/HwAgSysArbn/HwAgSysArbnPer1/HwAgArbn/VldtSnsrlsData/Pass ==
  In : Inport
  Action Port : ActionPort  ActionType=then
  CopyRight2 : Subsystem  Description=|  mask(Copyright Information){none=on}
      | Copyright info block.                                               
      |                                                                     
      | Place copyright information at the top of every subsystem in design.
      mask prompts: none "No parameters"
      mask help: Place copyright information at the top of every subsystem in design.
      mask Display:
      | NxtrConf = 'Nexteer Confidential';
      | 
      | sys = bdroot; %handle for the current model ("system")
      | first = get_param(sys,'Created');
      | first = first(end-3:end);  %year is last four digits
      | 
      | last = get_param(sys,'LastModifiedDate');
      | if isempty(last)
      |     last = datestr(now,'yyyy');
      | else
      |     last = last(end-3:end);
      | end
      | 
      | if strcmp(first,last)
      |     fprintf('%s -- Copyright %s Nexteer',NxtrConf,first)
      | else
      |     fprintf('%s -- %s%s- %s Nexteer',NxtrConf,char(169),first,last)
      | end
  Out : Outport
  wires:
  In/1 -> Out/1

== system SF045A_HwAgSysArbn/HwAgSysArbn/HwAgSysArbnPer1/HwAgArbn/VldtSnsrlsData/ThdExcdd ==
  Action Port : ActionPort  ActionType=else
  Constant1 : Constant  RequirementInfo={} %GIDa_d0c90f58_16bd_441d_9f25_306945bdc86c  Value=0
  Constant2 : Constant  RequirementInfo={} %GIDa_80a4bd6b_66bb_466e_92fd_268653573d1f  Value=NODEBSTEP_CNT_U16
  Constant3 : Constant  RequirementInfo={} %GIDa_b869d25f_3332_482d_b6cc_f4cf8728ad4e  Value=HwAgSnsrlsThdExcdd
  CopyRight2 : Subsystem  Description=|  mask(Copyright Information){none=on}
      | Copyright info block.                                               
      |                                                                     
      | Place copyright information at the top of every subsystem in design.
      mask prompts: none "No parameters"
      mask help: Place copyright information at the top of every subsystem in design.
      mask Display:
      | NxtrConf = 'Nexteer Confidential';
      | 
      | sys = bdroot; %handle for the current model ("system")
      | first = get_param(sys,'Created');
      | first = first(end-3:end);  %year is last four digits
      | 
      | last = get_param(sys,'LastModifiedDate');
      | if isempty(last)
      |     last = datestr(now,'yyyy');
      | else
      |     last = last(end-3:end);
      | end
      | 
      | if strcmp(first,last)
      |     fprintf('%s -- Copyright %s Nexteer',NxtrConf,first)
      | else
      |     fprintf('%s -- %s%s- %s Nexteer',NxtrConf,char(169),first,last)
      | end
  Data Store Write3 : DataStoreWrite  RequirementInfo={} %GIDa_41ac5734_6613_430d_bc30_5d7926b08b3d  DataStoreName=HwAgKineFlt
  Enumerated Constant1 : simulink/Sources/Enumerated Constant  RequirementInfo={} %GIDa_5018205c_7889_4e2b_9729_3068da7db44b  OutDataTypeStr=Enum: NtcSts1  Value=NtcSts1.NTCSTS_FAILD  SampleTime=inf
  Kinematic Integrity : Subsystem  RequirementInfo={} %GIDa_51e49fb6_28b4_4575_9520_9187071930dd  mask(SetNTC){}
      mask help: SetNTC library block
  SET1 : Constant  Value=0  OutDataTypeStr=single
      settings: AttributesFormatString=%<OutDataTypeStr>
  SET2 : Constant  Value=true  OutDataTypeStr=boolean
      settings: AttributesFormatString=%<OutDataTypeStr>
  Out : Outport
  wires:
  Enumerated Constant1/1 -> Kinematic Integrity/3(NtcSts)
  Constant1/1 -> Kinematic Integrity/2(NtcStInfo)
  Constant3/1 -> Kinematic Integrity/1(NtcNr)
  Constant2/1 -> Kinematic Integrity/4(DebStep)
  SET1/1 -> Out/1
  SET2/1 -> Data Store Write3/1

== system SF045A_HwAgSysArbn/HwAgSysArbn/HwAgSysArbnPer1/HwAgArbn/CalcHwAgCorrdConf /NoSensor/CopyRight2 ==

== system SF045A_HwAgSysArbn/HwAgSysArbn/HwAgSysArbnPer1/HwAgArbn/CalcHwAgCorrdConf /OneSensor/CopyRight2 ==

== system SF045A_HwAgSysArbn/HwAgSysArbn/HwAgSysArbnPer1/HwAgArbn/CalcHwAgCorrdConf /TwoSensors/CopyRight2 ==

== system SF045A_HwAgSysArbn/HwAgSysArbn/HwAgSysArbnPer1/HwAgArbn/CalcHwAgCorrdConf /Zero/CopyRight2 ==

== system SF045A_HwAgSysArbn/HwAgSysArbn/HwAgSysArbnPer1/HwAgArbn/CalcPinionVel/MotorVelocityVld/CopyRight2 ==

== system SF045A_HwAgSysArbn/HwAgSysArbn/HwAgSysArbnPer1/HwAgArbn/CalcPinionVel/MotorVelocityVld/TbarVelocity ==
  HwTq : Inport  RequirementInfo={} %GIDa_0c94317e_84e4_4818_ad29_483b48c9fa20
  Add2 : Sum  RequirementInfo="{'linktype_rmi_doors' '00012ce0 (/E-STEER Core/SubSystem Specifications/Application Functions - EA4/SF045A Handwheel Angle System Arbitration)' '#SF045A_137' 'true' 'REQ:  SF045A_137' '' } %GIDa_d3c9e154_9d80_451d_8f2c_aa0e85945f83"  Inputs=+-
  Constant1 : Constant  RequirementInfo="{'linktype_rmi_doors' '00012ce0 (/E-STEER Core/SubSystem Specifications/Application Functions - EA4/SF045A Handwheel Angle System Arbitration)' '#SF045A_137' 'true' 'REQ:  SF045A_137' '' } %GIDa_df013f6c_795c_45bc_8be7_40feab5d7712"  Value=ARCHGLBPRM_PIOVER180_ULS_F32
  CopyRight2 : Subsystem  Description=|  mask(Copyright Information){none=on}
      | Copyright info block.                                               
      |                                                                     
      | Place copyright information at the top of every subsystem in design.
      mask prompts: none "No parameters"
      mask help: Place copyright information at the top of every subsystem in design.
      mask Display:
      | NxtrConf = 'Nexteer Confidential';
      | 
      | sys = bdroot; %handle for the current model ("system")
      | first = get_param(sys,'Created');
      | first = first(end-3:end);  %year is last four digits
      | 
      | last = get_param(sys,'LastModifiedDate');
      | if isempty(last)
      |     last = datestr(now,'yyyy');
      | else
      |     last = last(end-3:end);
      | end
      | 
      | if strcmp(first,last)
      |     fprintf('%s -- Copyright %s Nexteer',NxtrConf,first)
      | else
      |     fprintf('%s -- %s%s- %s Nexteer',NxtrConf,char(169),first,last)
      | end
  Data Store Read : DataStoreRead  RequirementInfo="{'linktype_rmi_doors' '00012ce0 (/E-STEER Core/SubSystem Specifications/Application Functions - EA4/SF045A Handwheel Angle System Arbitration)' '#SF045A_137' 'true' 'REQ:  SF045A_137' '' } %GIDa_47707930_7442_43e8_9811_4a9456378cfe"  Priority=1  DataStoreName=TqSnsrAgPrev
      settings: AttributesFormatString=Priority%<priority>
  Data Store Write : DataStoreWrite  RequirementInfo="{'linktype_rmi_doors' '00012ce0 (/E-STEER Core/SubSystem Specifications/Application Functions - EA4/SF045A Handwheel Angle System Arbitration)' '#SF045A_137' 'true' 'REQ:  SF045A_137' '' } %GIDa_fd872182_71a5_47b5_95aa_492fcd71db48"  Priority=2  DataStoreName=TqSnsrAgPrev
      settings: AttributesFormatString=priority %<Priority>
  Divide : Product  RequirementInfo="{'linktype_rmi_doors' '00012ce0 (/E-STEER Core/SubSystem Specifications/Application Functions - EA4/SF045A Handwheel Angle System Arbitration)' '#SF045A_137' 'true' 'REQ:  SF045A_137' '' } %GIDa_f210fab7_58a3_47d7_ad14_aac231e9cef6"  Inputs=*/
  Divide1 : Product  RequirementInfo="{'linktype_rmi_doors' '00012ce0 (/E-STEER Core/SubSystem Specifications/Application Functions - EA4/SF045A Handwheel Angle System Arbitration)' '#SF045A_137' 'true' 'REQ:  SF045A_137' '' } %GIDa_dd9f0223_1ced_4312_89e1_2ec98aa7b75a"  Inputs=*/
  FilLpUpdOutp : Fil/FilLpUpdOutp  RequirementInfo="{'linktype_rmi_doors' '00012ce0 (/E-STEER Core/SubSystem Specifications/Application Functions - EA4/SF045A Handwheel Angle System Arbitration)' '#SF045A_137' 'true' 'REQ:  SF045A_137' '' } %GIDa_84595fec_2794_4e82_93b6_088276f1824d"  StVar=TqSnsrVelFil
      settings: AttributesFormatString=StVar: %<StVar>
  LoopTime1 : Constant  RequirementInfo="{'linktype_rmi_doors' '00012ce0 (/E-STEER Core/SubSystem Specifications/Application Functions - EA4/SF045A Handwheel Angle System Arbitration)' '#SF045A_137' 'true' 'REQ:  SF045A_137' '' } %GIDa_1b0a4283_ba13_411f_9403_75bc769a4ed8"  Value=ARCHGLBPRM_2MILLISEC_SEC_F32
  Mult2 : Product  RequirementInfo="{'linktype_rmi_doors' '00012ce0 (/E-STEER Core/SubSystem Specifications/Application Functions - EA4/SF045A Handwheel Angle System Arbitration)' '#SF045A_137' 'true' 'REQ:  SF045A_137' '' } %GIDa_0277f8c5_eeaf_4ea8_b3ac_7f92af0b651c"  Inputs=**
  k_S_TbarStiff_NmpDeg_u9p7 : Constant  RequirementInfo="{'linktype_rmi_doors' '00012ce0 (/E-STEER Core/SubSystem Specifications/Application Functions - EA4/SF045A Handwheel Angle System Arbitration)' '#SF045A_137' 'true' 'REQ:  SF045A_137' '' } %GIDa_e3201b7c_dcab_4eb3_8a76_96d543e4a14e"  Value=SysGlbPrmTorsBarStfn
  TbarVel : Outport
  wires:
  HwTq/1 -> Divide/1
  k_S_TbarStiff_NmpDeg_u9p7/1 -> Divide/2
  Divide/1 -> Add2/1, Data Store Write/1
  Divide1/1 -> FilLpUpdOutp/1
  FilLpUpdOutp/1 -> Mult2/1
  Add2/1 -> Divide1/1
  LoopTime1/1 -> Divide1/2
  Data Store Read/1 -> Add2/2
  Constant1/1 -> Mult2/2
  Mult2/1 -> TbarVel/1

== system SF045A_HwAgSysArbn/HwAgSysArbn/HwAgSysArbnPer1/HwAgArbn/CalcPinionVel/PinionAnglegConf/CopyRight2 ==
